simulink model "rds_modul"  (R2017a)
settings: Solver=FixedStepAuto  StartTime=-0.016  StopTime=0.016  FixedStep=4.210526315789473e-06  MaxStep=4.210526315789473e-06  RelTol=1e-3
libraries: dspsrcs4 x5, commsrccod2 x1, dspsigops x1, commfilt2 x1, commrandsrc3 x1
settings Model: Creator=SPA  LastModifiedBy=SPA

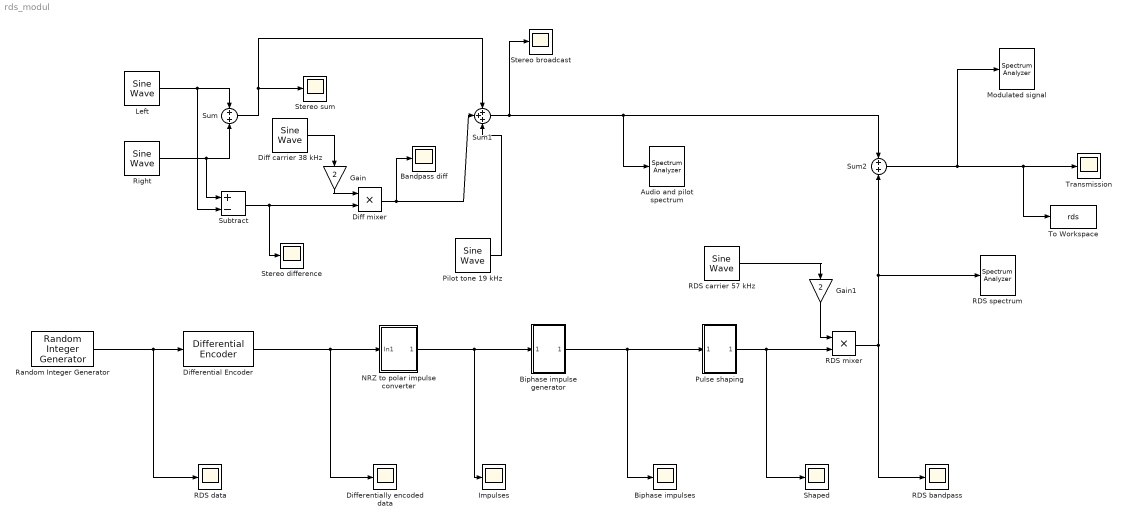
== system rds_modul ==
  Audio and pilot spectrum : SpectrumAnalyzer
  Bandpass diff : Scope
  Biphase impulse generator : Subsystem
  Biphase impulses : Scope
  Diff carrier 38 kHz : dspsrcs4/Sine Wave  Amplitude=1  Frequency=38000  Phase=pi/2  SampleMode=Discrete  OutComplex=Real  CompMethod=Trigonometric fcn  TableSize=Speed  SampleTime=4.210526315789473e-06  SamplesPerFrame=7600  ResetState=Restart at time zero  OutputFrames=off  dataType=double  wordLen=16  udDataType=sfix(16)  fracBitsMode=Best precision  numFracBits=15  OutDataTypeStr=double  LastOutDataTypeStr=double
  Diff mixer : Product
  Differential Encoder : commsrccod2/Differential Encoder  InitCond=0
      settings: SourceProductName=Communications System Toolbox  SourceProductBaseCode=CM
  "Differentially encoded data " : Scope
  Gain : Gain  Gain=2
  Gain1 : Gain  Gain=2
  Impulses : Scope
  Left : dspsrcs4/Sine Wave  Amplitude=1  Frequency=1000  Phase=0  SampleMode=Discrete  OutComplex=Real  CompMethod=Trigonometric fcn  TableSize=Speed  SampleTime=4.210526315789473e-06  SamplesPerFrame=7600  ResetState=Restart at time zero  OutputFrames=off  dataType=double  wordLen=16  udDataType=sfix(16)  fracBitsMode=Best precision  numFracBits=15  OutDataTypeStr=double  LastOutDataTypeStr=double
  Modulated signal : SpectrumAnalyzer
  NRZ to polar impulse converter : Subsystem
  "Pilot tone 19 kHz " : dspsrcs4/Sine Wave  Amplitude=1  Frequency=19000  Phase=pi/2  SampleMode=Discrete  OutComplex=Real  CompMethod=Trigonometric fcn  TableSize=Speed  SampleTime=4.210526315789473e-06  SamplesPerFrame=7600  ResetState=Restart at time zero  OutputFrames=off  dataType=double  wordLen=16  udDataType=sfix(16)  fracBitsMode=Best precision  numFracBits=15  OutDataTypeStr=double  LastOutDataTypeStr=double
  Pulse shaping : Subsystem
  RDS bandpass : Scope
  RDS carrier 57 kHz : dspsrcs4/Sine Wave  Amplitude=1  Frequency=57000  Phase=pi/2  SampleMode=Discrete  OutComplex=Real  CompMethod=Trigonometric fcn  TableSize=Speed  SampleTime=4.210526315789473e-06  SamplesPerFrame=7600  ResetState=Restart at time zero  OutputFrames=off  dataType=double  wordLen=16  udDataType=sfix(16)  fracBitsMode=Best precision  numFracBits=15  OutDataTypeStr=double  LastOutDataTypeStr=double
  "RDS data " : Scope
  RDS mixer : Product
  RDS spectrum : SpectrumAnalyzer
  Random Integer Generator : commrandsrc3/Random Integer Generator  SetSize=2  SeedSource=Auto  Seed=0  SampleTime=8.421052631578947e-04  SamplesPerFrame=38  OutputDataType=double  SimulateUsing=Interpreted execution
  "Right " : dspsrcs4/Sine Wave  Amplitude=1  Frequency=1000  Phase=pi/2  SampleMode=Discrete  OutComplex=Real  CompMethod=Trigonometric fcn  TableSize=Speed  SampleTime=4.210526315789473e-06  SamplesPerFrame=7600  ResetState=Restart at time zero  OutputFrames=off  dataType=double  wordLen=16  udDataType=sfix(16)  fracBitsMode=Best precision  numFracBits=15  OutDataTypeStr=double  LastOutDataTypeStr=double
  "Shaped " : Scope
  Stereo broadcast : Scope
  Stereo difference : Scope
  Stereo sum : Scope
  Subtract : Sum  Inputs=+-
  Sum : Sum  Inputs=2
  Sum1 : Sum  Inputs=3
  Sum2 : Sum  Inputs=2
  To Workspace : ToWorkspace  VariableName=rds  SaveFormat=Timeseries  SampleTime=-1
  Transmission : Scope
  wires:
  "Right "/1 -> Subtract/1, Sum/2
  Left/1 -> Subtract/2, Sum/1
  Subtract/1 -> Diff mixer/2, Stereo difference/1
  Diff mixer/1 -> Bandpass diff/1, Sum1/2
  "Pilot tone 19 kHz "/1 -> Sum1/3
  Sum1/1 -> Audio and pilot spectrum/1, Sum2/1, Stereo broadcast/1
  Sum2/1 -> Modulated signal/1, To Workspace/1, Transmission/1
  Sum/1 -> Sum1/1, Stereo sum/1
  Diff carrier 38 kHz/1 -> Gain/1
  RDS mixer/1 -> RDS bandpass/1, Sum2/2, RDS spectrum/1
  RDS carrier 57 kHz/1 -> Gain1/1
  Differential Encoder/1 -> NRZ to polar impulse converter/1(In1), "Differentially encoded data "/1
  Random Integer Generator/1 -> "RDS data "/1, Differential Encoder/1
  Biphase impulse generator/1(Out1) -> Pulse shaping/1(In1), Biphase impulses/1
  Pulse shaping/1(Out1) -> RDS mixer/2, "Shaped "/1
  NRZ to polar impulse converter/1(Out1) -> Impulses/1, Biphase impulse generator/1(In1)
  Gain/1 -> Diff mixer/1
  Gain1/1 -> RDS mixer/1

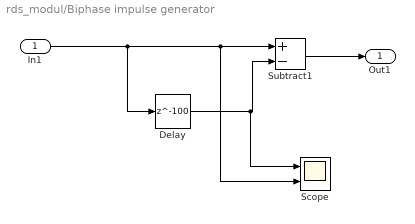
== system rds_modul/Biphase impulse generator ==
  In1 : Inport
  Delay : Delay  DelayLength=100  InitialCondition=0  InputProcessing=Columns as channels (frame based)
  Scope : Scope  NumInputPorts=2
  Subtract1 : Sum  Inputs=+-
  Out1 : Outport
  wires:
  Delay/1 -> Scope/1, Subtract1/2
  Subtract1/1 -> Out1/1
  In1/1 -> Scope/2, Subtract1/1, Delay/1

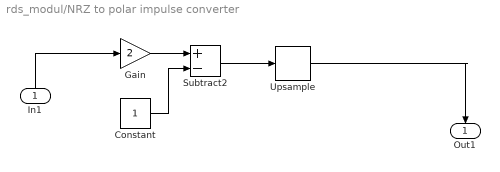
== system rds_modul/NRZ to polar impulse converter ==
  In1 : Inport
  Constant : Constant
  Gain : Gain  Gain=2
  Subtract2 : Sum  Inputs=+-
  Upsample : dspsigops/Upsample  N=200  phase=0  InputProcessing=Columns as channels (frame based)  RateOptions=Enforce single-rate processing  ic=0  mode=Unused parameter value
  Out1 : Outport
  wires:
  Gain/1 -> Subtract2/1
  Constant/1 -> Subtract2/2
  In1/1 -> Gain/1
  Subtract2/1 -> Upsample/1
  Upsample/1 -> Out1/1

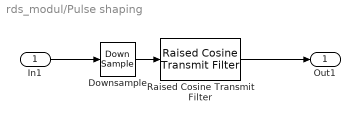
== system rds_modul/Pulse shaping ==
  In1 : Inport
  Downsample : DownSample  N=100
  Raised Cosine Transmit Filter : commfilt2/Raised Cosine Transmit Filter  filtType=Square root  R=1  filtSpan=76  N=100  filterGain=1  InputProcessing=Columns as channels (frame based)  RateOptions=Enforce single-rate processing  framing=Mute  checkCoeff=off  variableName=rcTxFilt  checkGain=Normalized  sampMode=Mute  saveAsFlag=0  currentFiltSpan=76  D=(76)/2  launchFVT=on  roundingMode=Floor  overflowMode=off  coeffDataTypeStr=Inherit: Same word length as input  coeffMin=[]  coeffMax=[]  coeffLastDataTypeStr=Inherit: Same word length as input  outputDataTypeStr=Inherit: Same as accumulator  outputMin=[]  outputMax=[]  outputLastDataTypeStr=Inherit: Same as accumulator
  Out1 : Outport
  wires:
  In1/1 -> Downsample/1
  Raised Cosine Transmit Filter/1 -> Out1/1
  Downsample/1 -> Raised Cosine Transmit Filter/1
